simulink model "Arm_core_design_block"  (R2021a)
settings: Solver=VariableStepAuto  StartTime=0.0  StopTime=500  RelTol=1e-3
undefined symbols (not defined in the file or in its folder): AXI4, Lite
libraries: hdlBasic x907, xbsIndex_r4 x1
(part 3 of 7)

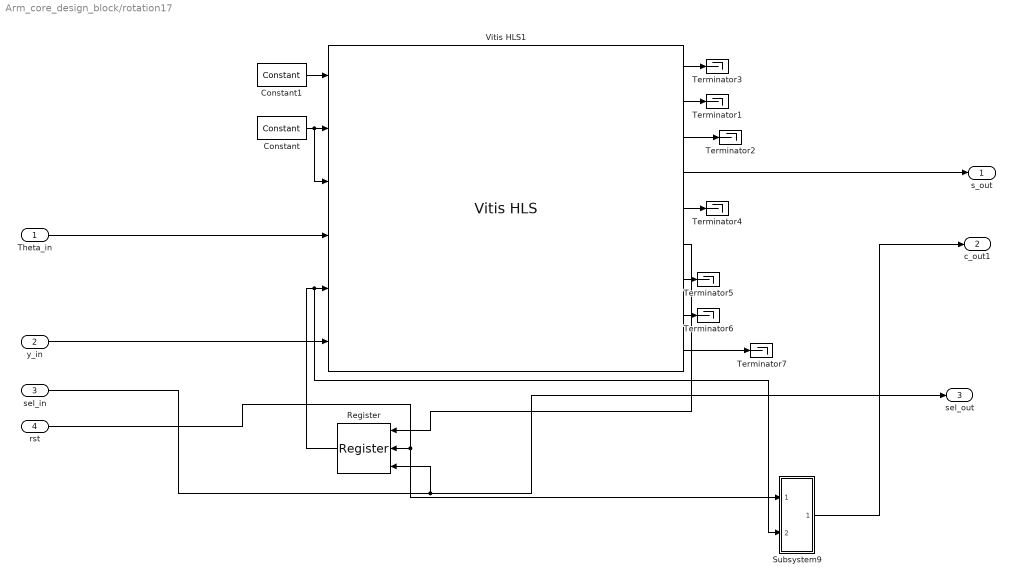
== system Arm_core_design_block/rotation17 ==
  Theta_in : Inport
  y_in : Inport  Port=2
  sel_in : Inport  Port=3
  rst : Inport  Port=4
  Constant : hdlBasic/Constant  const=1.0  gui_display_data_type=Boolean  arith_type=Boolean  n_bits=16  bin_pt=14  preci_type=Single  exp_width=8  frac_width=24  explicit_period=off  period=1  XmcBlockStatus=1  maskContainerNames=tabcontainer1  block_type=constant  block_config=sysgen:Constant_config
  Constant1 : hdlBasic/Constant  const=0  gui_display_data_type=Boolean  arith_type=Boolean  n_bits=16  bin_pt=14  preci_type=Single  exp_width=8  frac_width=24  explicit_period=off  period=1  XmcBlockStatus=1  maskContainerNames=tabcontainer1  block_type=constant  block_config=sysgen:Constant_config
  Register : hdlBasic/Register  init=0  rst=on  en=on  XmcBlockStatus=1  maskContainerNames=tabcontainer1  block_type=register  block_config=sysgen:Register_config
  Subsystem9 : Subsystem
  Terminator{1..7} (7 alike) : Terminator
  Vitis HLS1 : hdlBasic/Vitis HLS  anytable='.\cordic_proj5\solution1'  fast_sim=off  display_datatype=off  rate_propagation_method=Simulink system period  model_file_path=''  latency=1  block_type=vitis_hls
      settings: infoedit=This block allows including C,C++ and SystemC source files in System Generator for DSP designs.
  s_out : Outport
  c_out1 : Outport  Port=2
  sel_out : Outport  Port=3
  wires:
  Constant1/1 -> Vitis HLS1/1
  Vitis HLS1/6 -> Register/1
  y_in/1 -> Vitis HLS1/6
  Constant/1 -> Vitis HLS1/3, Vitis HLS1/2
  Vitis HLS1/4 -> s_out/1
  Theta_in/1 -> Vitis HLS1/4
  sel_in/1 -> sel_out/1, Register/3
  Vitis HLS1/1 -> Terminator3/1
  Vitis HLS1/2 -> Terminator1/1
  Vitis HLS1/3 -> Terminator2/1
  Vitis HLS1/5 -> Terminator4/1
  Vitis HLS1/7 -> Terminator5/1
  Vitis HLS1/8 -> Terminator6/1
  Vitis HLS1/9 -> Terminator7/1
  Register/1 -> Subsystem9/2(reg_i), Vitis HLS1/5
  rst/1 -> Subsystem9/1(rst), Register/2
  Subsystem9/1(reg_o) -> c_out1/1

== system Arm_core_design_block/rotation19 ==
  Theta_in : Inport
  y_in : Inport  Port=2
  rst : Inport  Port=3
  Constant : hdlBasic/Constant  const=1.0  gui_display_data_type=Boolean  arith_type=Boolean  n_bits=16  bin_pt=14  preci_type=Single  exp_width=8  frac_width=24  explicit_period=off  period=1  XmcBlockStatus=1  maskContainerNames=tabcontainer1  block_type=constant  block_config=sysgen:Constant_config
  Constant1 : hdlBasic/Constant  const=0  gui_display_data_type=Boolean  arith_type=Boolean  n_bits=16  bin_pt=14  preci_type=Single  exp_width=8  frac_width=24  explicit_period=off  period=1  XmcBlockStatus=1  maskContainerNames=tabcontainer1  block_type=constant  block_config=sysgen:Constant_config
  Register : hdlBasic/Register  init=0  rst=on  en=on  XmcBlockStatus=1  maskContainerNames=tabcontainer1  block_type=register  block_config=sysgen:Register_config
  Subsystem9 : Subsystem
  Terminator{1..6} (6 alike) : Terminator
  Vitis HLS1 : hdlBasic/Vitis HLS  anytable='.\cordic_proj5\solution1'  fast_sim=off  display_datatype=off  rate_propagation_method=Simulink system period  model_file_path=''  latency=1  block_type=vitis_hls
      settings: infoedit=This block allows including C,C++ and SystemC source files in System Generator for DSP designs.
  s_out : Outport
  c_out1 : Outport  Port=2
  sel_out : Outport  Port=3
  wires:
  Constant1/1 -> Vitis HLS1/1
  Vitis HLS1/6 -> Register/1
  y_in/1 -> Vitis HLS1/6
  Constant/1 -> Vitis HLS1/3, Vitis HLS1/2
  Vitis HLS1/7 -> sel_out/1, Register/3
  Vitis HLS1/4 -> s_out/1
  Theta_in/1 -> Vitis HLS1/4
  Vitis HLS1/1 -> Terminator3/1
  Vitis HLS1/2 -> Terminator1/1
  Vitis HLS1/5 -> Terminator2/1
  Vitis HLS1/8 -> Terminator5/1
  Vitis HLS1/9 -> Terminator4/1
  Vitis HLS1/3 -> Terminator6/1
  rst/1 -> Subsystem9/1(rst), Register/2
  Register/1 -> Subsystem9/2(reg_i), Vitis HLS1/5
  Subsystem9/1(reg_o) -> c_out1/1

== system Arm_core_design_block/rotation2 ==
  Theta_in : Inport
  y_in : Inport  Port=2
  rst : Inport  Port=3
  Constant : hdlBasic/Constant  const=1.0  gui_display_data_type=Boolean  arith_type=Boolean  n_bits=16  bin_pt=14  preci_type=Single  exp_width=8  frac_width=24  explicit_period=off  period=1  XmcBlockStatus=1  maskContainerNames=tabcontainer1  block_type=constant  block_config=sysgen:Constant_config
  Constant1 : hdlBasic/Constant  const=0  gui_display_data_type=Boolean  arith_type=Boolean  n_bits=16  bin_pt=14  preci_type=Single  exp_width=8  frac_width=24  explicit_period=off  period=1  XmcBlockStatus=1  maskContainerNames=tabcontainer1  block_type=constant  block_config=sysgen:Constant_config
  Register : hdlBasic/Register  init=0  rst=on  en=on  XmcBlockStatus=1  maskContainerNames=tabcontainer1  block_type=register  block_config=sysgen:Register_config
  Terminator{1..6} (6 alike) : Terminator
  Vitis HLS1 : hdlBasic/Vitis HLS  anytable='.\cordic_proj5\solution1'  fast_sim=off  display_datatype=off  rate_propagation_method=Simulink system period  model_file_path=''  latency=1  block_type=vitis_hls
      settings: infoedit=This block allows including C,C++ and SystemC source files in System Generator for DSP designs.
  s_out : Outport
  c_out1 : Outport  Port=2
  sel_out : Outport  Port=3
  wires:
  Constant1/1 -> Vitis HLS1/1
  Vitis HLS1/6 -> Register/1
  y_in/1 -> Vitis HLS1/6
  Constant/1 -> Vitis HLS1/3, Vitis HLS1/2
  Vitis HLS1/7 -> sel_out/1, Register/3
  Vitis HLS1/4 -> s_out/1
  Theta_in/1 -> Vitis HLS1/4
  Vitis HLS1/1 -> Terminator3/1
  Vitis HLS1/2 -> Terminator1/1
  Vitis HLS1/5 -> Terminator2/1
  Vitis HLS1/8 -> Terminator5/1
  Vitis HLS1/9 -> Terminator4/1
  Vitis HLS1/3 -> Terminator6/1
  rst/1 -> Register/2
  Register/1 -> c_out1/1, Vitis HLS1/5

== system Arm_core_design_block/rotation3 ==
  Theta_in : Inport
  y_in : Inport  Port=2
  sel_in : Inport  Port=3
  rst : Inport  Port=4
  Constant : hdlBasic/Constant  const=1.0  gui_display_data_type=Boolean  arith_type=Boolean  n_bits=16  bin_pt=14  preci_type=Single  exp_width=8  frac_width=24  explicit_period=off  period=1  XmcBlockStatus=1  maskContainerNames=tabcontainer1  block_type=constant  block_config=sysgen:Constant_config
  Constant1 : hdlBasic/Constant  const=0  gui_display_data_type=Boolean  arith_type=Boolean  n_bits=16  bin_pt=14  preci_type=Single  exp_width=8  frac_width=24  explicit_period=off  period=1  XmcBlockStatus=1  maskContainerNames=tabcontainer1  block_type=constant  block_config=sysgen:Constant_config
  Register : hdlBasic/Register  init=0  rst=on  en=on  XmcBlockStatus=1  maskContainerNames=tabcontainer1  block_type=register  block_config=sysgen:Register_config
  Terminator{1..7} (7 alike) : Terminator
  Vitis HLS1 : hdlBasic/Vitis HLS  anytable='.\cordic_proj5\solution1'  fast_sim=off  display_datatype=off  rate_propagation_method=Simulink system period  model_file_path=''  latency=1  block_type=vitis_hls
      settings: infoedit=This block allows including C,C++ and SystemC source files in System Generator for DSP designs.
  s_out : Outport
  c_out1 : Outport  Port=2
  wires:
  Constant1/1 -> Vitis HLS1/1
  y_in/1 -> Vitis HLS1/6
  Constant/1 -> Vitis HLS1/3, Vitis HLS1/2
  Vitis HLS1/4 -> s_out/1
  Theta_in/1 -> Vitis HLS1/4
  sel_in/1 -> Register/3
  Vitis HLS1/1 -> Terminator3/1
  Vitis HLS1/2 -> Terminator1/1
  Vitis HLS1/3 -> Terminator2/1
  Vitis HLS1/5 -> Terminator4/1
  Vitis HLS1/7 -> Terminator5/1
  Vitis HLS1/8 -> Terminator6/1
  Vitis HLS1/9 -> Terminator7/1
  rst/1 -> Register/2
  Vitis HLS1/6 -> Register/1
  Register/1 -> c_out1/1, Vitis HLS1/5

== system Arm_core_design_block/rotation4 ==
  Theta_in : Inport
  y_in : Inport  Port=2
  rst : Inport  Port=3
  Constant : hdlBasic/Constant  const=1.0  gui_display_data_type=Boolean  arith_type=Boolean  n_bits=16  bin_pt=14  preci_type=Single  exp_width=8  frac_width=24  explicit_period=off  period=1  XmcBlockStatus=1  maskContainerNames=tabcontainer1  block_type=constant  block_config=sysgen:Constant_config
  Constant1 : hdlBasic/Constant  const=0  gui_display_data_type=Boolean  arith_type=Boolean  n_bits=16  bin_pt=14  preci_type=Single  exp_width=8  frac_width=24  explicit_period=off  period=1  XmcBlockStatus=1  maskContainerNames=tabcontainer1  block_type=constant  block_config=sysgen:Constant_config
  Register : hdlBasic/Register  init=0  rst=on  en=on  XmcBlockStatus=1  maskContainerNames=tabcontainer1  block_type=register  block_config=sysgen:Register_config
  Terminator{1..6} (6 alike) : Terminator
  Vitis HLS1 : hdlBasic/Vitis HLS  anytable='.\cordic_proj5\solution1'  fast_sim=off  display_datatype=off  rate_propagation_method=Simulink system period  model_file_path=''  latency=1  block_type=vitis_hls
      settings: infoedit=This block allows including C,C++ and SystemC source files in System Generator for DSP designs.
  s_out : Outport
  c_out1 : Outport  Port=2
  sel_out : Outport  Port=3
  wires:
  Constant1/1 -> Vitis HLS1/1
  Vitis HLS1/6 -> Register/1
  y_in/1 -> Vitis HLS1/6
  Constant/1 -> Vitis HLS1/3, Vitis HLS1/2
  Vitis HLS1/7 -> sel_out/1, Register/3
  Vitis HLS1/4 -> s_out/1
  Theta_in/1 -> Vitis HLS1/4
  Vitis HLS1/1 -> Terminator3/1
  Vitis HLS1/2 -> Terminator1/1
  Vitis HLS1/5 -> Terminator2/1
  Vitis HLS1/8 -> Terminator5/1
  Vitis HLS1/9 -> Terminator4/1
  Vitis HLS1/3 -> Terminator6/1
  rst/1 -> Register/2
  Register/1 -> c_out1/1, Vitis HLS1/5

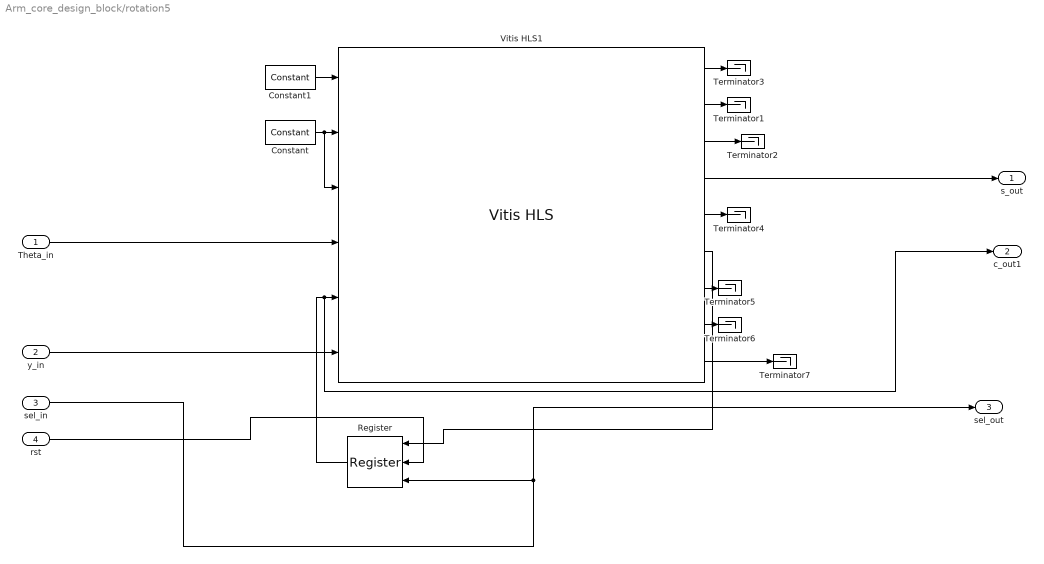
== system Arm_core_design_block/rotation5 ==
  Theta_in : Inport
  y_in : Inport  Port=2
  sel_in : Inport  Port=3
  rst : Inport  Port=4
  Constant : hdlBasic/Constant  const=1.0  gui_display_data_type=Boolean  arith_type=Boolean  n_bits=16  bin_pt=14  preci_type=Single  exp_width=8  frac_width=24  explicit_period=off  period=1  XmcBlockStatus=1  maskContainerNames=tabcontainer1  block_type=constant  block_config=sysgen:Constant_config
  Constant1 : hdlBasic/Constant  const=0  gui_display_data_type=Boolean  arith_type=Boolean  n_bits=16  bin_pt=14  preci_type=Single  exp_width=8  frac_width=24  explicit_period=off  period=1  XmcBlockStatus=1  maskContainerNames=tabcontainer1  block_type=constant  block_config=sysgen:Constant_config
  Register : hdlBasic/Register  init=0  rst=on  en=on  XmcBlockStatus=1  maskContainerNames=tabcontainer1  block_type=register  block_config=sysgen:Register_config
  Terminator{1..7} (7 alike) : Terminator
  Vitis HLS1 : hdlBasic/Vitis HLS  anytable='.\cordic_proj5\solution1'  fast_sim=off  display_datatype=off  rate_propagation_method=Simulink system period  model_file_path=''  latency=1  block_type=vitis_hls
      settings: infoedit=This block allows including C,C++ and SystemC source files in System Generator for DSP designs.
  s_out : Outport
  c_out1 : Outport  Port=2
  sel_out : Outport  Port=3
  wires:
  Constant1/1 -> Vitis HLS1/1
  Vitis HLS1/6 -> Register/1
  y_in/1 -> Vitis HLS1/6
  Constant/1 -> Vitis HLS1/3, Vitis HLS1/2
  Vitis HLS1/4 -> s_out/1
  Theta_in/1 -> Vitis HLS1/4
  sel_in/1 -> sel_out/1, Register/3
  Vitis HLS1/1 -> Terminator3/1
  Vitis HLS1/2 -> Terminator1/1
  Vitis HLS1/3 -> Terminator2/1
  Vitis HLS1/5 -> Terminator4/1
  Vitis HLS1/7 -> Terminator5/1
  Vitis HLS1/8 -> Terminator6/1
  Vitis HLS1/9 -> Terminator7/1
  Register/1 -> c_out1/1, Vitis HLS1/5
  rst/1 -> Register/2

== system Arm_core_design_block/rotation6 ==
  Theta_in : Inport
  y_in : Inport  Port=2
  sel_in : Inport  Port=3
  rst : Inport  Port=4
  Constant : hdlBasic/Constant  const=1.0  gui_display_data_type=Boolean  arith_type=Boolean  n_bits=16  bin_pt=14  preci_type=Single  exp_width=8  frac_width=24  explicit_period=off  period=1  XmcBlockStatus=1  maskContainerNames=tabcontainer1  block_type=constant  block_config=sysgen:Constant_config
  Constant1 : hdlBasic/Constant  const=0  gui_display_data_type=Boolean  arith_type=Boolean  n_bits=16  bin_pt=14  preci_type=Single  exp_width=8  frac_width=24  explicit_period=off  period=1  XmcBlockStatus=1  maskContainerNames=tabcontainer1  block_type=constant  block_config=sysgen:Constant_config
  Register : hdlBasic/Register  init=0  rst=on  en=on  XmcBlockStatus=1  maskContainerNames=tabcontainer1  block_type=register  block_config=sysgen:Register_config
  Register1 : hdlBasic/Register  init=0  rst=on  en=on  XmcBlockStatus=1  maskContainerNames=tabcontainer1  block_type=register  block_config=sysgen:Register_config
  Terminator{1..7} (7 alike) : Terminator
  Vitis HLS1 : hdlBasic/Vitis HLS  anytable='.\cordic_proj5\solution1'  fast_sim=off  display_datatype=off  rate_propagation_method=Simulink system period  model_file_path=''  latency=1  block_type=vitis_hls
      settings: infoedit=This block allows including C,C++ and SystemC source files in System Generator for DSP designs.
  s_out : Outport
  c_out1 : Outport  Port=2
  wires:
  Constant1/1 -> Vitis HLS1/1
  y_in/1 -> Vitis HLS1/6
  Constant/1 -> Vitis HLS1/3, Vitis HLS1/2
  Vitis HLS1/4 -> Register1/1
  Theta_in/1 -> Vitis HLS1/4
  sel_in/1 -> Register1/3, Register/3
  Vitis HLS1/1 -> Terminator3/1
  Vitis HLS1/2 -> Terminator1/1
  Vitis HLS1/3 -> Terminator2/1
  Vitis HLS1/5 -> Terminator4/1
  Vitis HLS1/7 -> Terminator5/1
  Vitis HLS1/8 -> Terminator6/1
  Vitis HLS1/9 -> Terminator7/1
  rst/1 -> Register1/2, Register/2
  Register/1 -> c_out1/1, Vitis HLS1/5
  Vitis HLS1/6 -> Register/1
  Register1/1 -> s_out/1

== system Arm_core_design_block/rotation7 ==
  Theta_in : Inport
  y_in : Inport  Port=2
  rst : Inport  Port=3
  Constant : hdlBasic/Constant  const=1.0  gui_display_data_type=Boolean  arith_type=Boolean  n_bits=16  bin_pt=14  preci_type=Single  exp_width=8  frac_width=24  explicit_period=off  period=1  XmcBlockStatus=1  maskContainerNames=tabcontainer1  block_type=constant  block_config=sysgen:Constant_config
  Constant1 : hdlBasic/Constant  const=0  gui_display_data_type=Boolean  arith_type=Boolean  n_bits=16  bin_pt=14  preci_type=Single  exp_width=8  frac_width=24  explicit_period=off  period=1  XmcBlockStatus=1  maskContainerNames=tabcontainer1  block_type=constant  block_config=sysgen:Constant_config
  Register : hdlBasic/Register  init=0  rst=on  en=on  XmcBlockStatus=1  maskContainerNames=tabcontainer1  block_type=register  block_config=sysgen:Register_config
  Subsystem9 : Subsystem
  Terminator{1..6} (6 alike) : Terminator
  Vitis HLS1 : hdlBasic/Vitis HLS  anytable='.\cordic_proj5\solution1'  fast_sim=off  display_datatype=off  rate_propagation_method=Simulink system period  model_file_path=''  latency=1  block_type=vitis_hls
      settings: infoedit=This block allows including C,C++ and SystemC source files in System Generator for DSP designs.
  s_out : Outport
  c_out1 : Outport  Port=2
  sel_out : Outport  Port=3
  wires:
  Constant1/1 -> Vitis HLS1/1
  Vitis HLS1/6 -> Register/1
  y_in/1 -> Vitis HLS1/6
  Constant/1 -> Vitis HLS1/3, Vitis HLS1/2
  Vitis HLS1/7 -> sel_out/1, Register/3
  Vitis HLS1/4 -> s_out/1
  Theta_in/1 -> Vitis HLS1/4
  Vitis HLS1/1 -> Terminator3/1
  Vitis HLS1/2 -> Terminator1/1
  Vitis HLS1/5 -> Terminator2/1
  Vitis HLS1/8 -> Terminator5/1
  Vitis HLS1/9 -> Terminator4/1
  Vitis HLS1/3 -> Terminator6/1
  rst/1 -> Subsystem9/1(rst), Register/2
  Register/1 -> Subsystem9/2(reg_i), Vitis HLS1/5
  Subsystem9/1(reg_o) -> c_out1/1

== system Arm_core_design_block/rotation8 ==
  Theta_in : Inport
  y_in : Inport  Port=2
  rst : Inport  Port=3
  Constant : hdlBasic/Constant  const=1.0  gui_display_data_type=Boolean  arith_type=Boolean  n_bits=16  bin_pt=14  preci_type=Single  exp_width=8  frac_width=24  explicit_period=off  period=1  XmcBlockStatus=1  maskContainerNames=tabcontainer1  block_type=constant  block_config=sysgen:Constant_config
  Constant1 : hdlBasic/Constant  const=0  gui_display_data_type=Boolean  arith_type=Boolean  n_bits=16  bin_pt=14  preci_type=Single  exp_width=8  frac_width=24  explicit_period=off  period=1  XmcBlockStatus=1  maskContainerNames=tabcontainer1  block_type=constant  block_config=sysgen:Constant_config
  Register : hdlBasic/Register  init=0  rst=on  en=on  XmcBlockStatus=1  maskContainerNames=tabcontainer1  block_type=register  block_config=sysgen:Register_config
  Subsystem9 : Subsystem
  Terminator{1..6} (6 alike) : Terminator
  Vitis HLS1 : hdlBasic/Vitis HLS  anytable='.\cordic_proj5\solution1'  fast_sim=off  display_datatype=off  rate_propagation_method=Simulink system period  model_file_path=''  latency=1  block_type=vitis_hls
      settings: infoedit=This block allows including C,C++ and SystemC source files in System Generator for DSP designs.
  s_out : Outport
  c_out1 : Outport  Port=2
  sel_out : Outport  Port=3
  wires:
  Constant1/1 -> Vitis HLS1/1
  Vitis HLS1/6 -> Register/1
  y_in/1 -> Vitis HLS1/6
  Constant/1 -> Vitis HLS1/3, Vitis HLS1/2
  Vitis HLS1/7 -> sel_out/1, Register/3
  Vitis HLS1/4 -> s_out/1
  Theta_in/1 -> Vitis HLS1/4
  Vitis HLS1/1 -> Terminator3/1
  Vitis HLS1/2 -> Terminator1/1
  Vitis HLS1/5 -> Terminator2/1
  Vitis HLS1/8 -> Terminator5/1
  Vitis HLS1/9 -> Terminator4/1
  Vitis HLS1/3 -> Terminator6/1
  rst/1 -> Subsystem9/1(rst), Register/2
  Register/1 -> Subsystem9/2(reg_i), Vitis HLS1/5
  Subsystem9/1(reg_o) -> c_out1/1

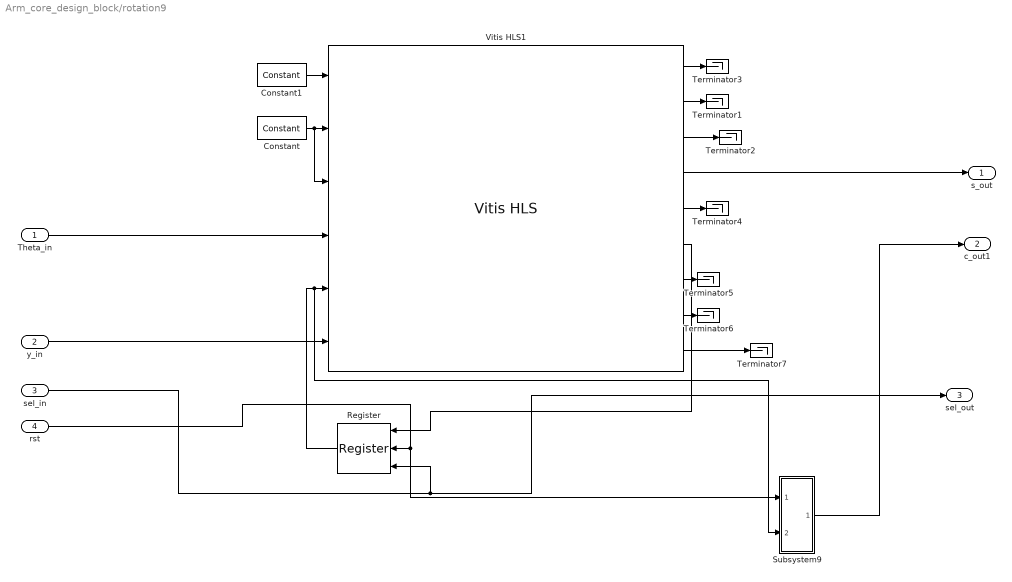
== system Arm_core_design_block/rotation9 ==
  Theta_in : Inport
  y_in : Inport  Port=2
  sel_in : Inport  Port=3
  rst : Inport  Port=4
  Constant : hdlBasic/Constant  const=1.0  gui_display_data_type=Boolean  arith_type=Boolean  n_bits=16  bin_pt=14  preci_type=Single  exp_width=8  frac_width=24  explicit_period=off  period=1  XmcBlockStatus=1  maskContainerNames=tabcontainer1  block_type=constant  block_config=sysgen:Constant_config
  Constant1 : hdlBasic/Constant  const=0  gui_display_data_type=Boolean  arith_type=Boolean  n_bits=16  bin_pt=14  preci_type=Single  exp_width=8  frac_width=24  explicit_period=off  period=1  XmcBlockStatus=1  maskContainerNames=tabcontainer1  block_type=constant  block_config=sysgen:Constant_config
  Register : hdlBasic/Register  init=0  rst=on  en=on  XmcBlockStatus=1  maskContainerNames=tabcontainer1  block_type=register  block_config=sysgen:Register_config
  Subsystem9 : Subsystem
  Terminator{1..7} (7 alike) : Terminator
  Vitis HLS1 : hdlBasic/Vitis HLS  anytable='.\cordic_proj5\solution1'  fast_sim=off  display_datatype=off  rate_propagation_method=Simulink system period  model_file_path=''  latency=1  block_type=vitis_hls
      settings: infoedit=This block allows including C,C++ and SystemC source files in System Generator for DSP designs.
  s_out : Outport
  c_out1 : Outport  Port=2
  sel_out : Outport  Port=3
  wires:
  Constant1/1 -> Vitis HLS1/1
  Vitis HLS1/6 -> Register/1
  y_in/1 -> Vitis HLS1/6
  Constant/1 -> Vitis HLS1/3, Vitis HLS1/2
  Vitis HLS1/4 -> s_out/1
  Theta_in/1 -> Vitis HLS1/4
  sel_in/1 -> sel_out/1, Register/3
  Vitis HLS1/1 -> Terminator3/1
  Vitis HLS1/2 -> Terminator1/1
  Vitis HLS1/3 -> Terminator2/1
  Vitis HLS1/5 -> Terminator4/1
  Vitis HLS1/7 -> Terminator5/1
  Vitis HLS1/8 -> Terminator6/1
  Vitis HLS1/9 -> Terminator7/1
  Register/1 -> Subsystem9/2(reg_i), Vitis HLS1/5
  rst/1 -> Subsystem9/1(rst), Register/2
  Subsystem9/1(reg_o) -> c_out1/1

== system Arm_core_design_block/Subsystem10/Subsystem10 ==
  reg_i : Inport
  Constant1 : hdlBasic/Constant  const=0  gui_display_data_type=Boolean  arith_type=Boolean  n_bits=16  bin_pt=1  preci_type=Single  exp_width=8  frac_width=24  explicit_period=off  period=1  XmcBlockStatus=1  maskContainerNames=tabcontainer1  block_type=constant  block_config=sysgen:Constant_config
  Mux1 : hdlBasic/Mux  inputs=2  en=off  latency=1  precision=Full  arith_type=Unsigned  n_bits=16  bin_pt=14  quantization=Truncate  overflow=Wrap  XmcBlockStatus=1  maskContainerNames=tabcontainer1  block_type=mux  block_config=sysgen:Mux_config
  Register2 : hdlBasic/Register  init=0  rst=off  en=off  XmcBlockStatus=1  maskContainerNames=tabcontainer1  block_type=register  block_config=sysgen:Register_config
  reg_o : Outport
  wires:
  reg_i/1 -> Register2/1, Mux1/2
  Mux1/1 -> reg_o/1
  Constant1/1 -> Mux1/3
  Register2/1 -> Mux1/1

== system Arm_core_design_block/Subsystem10/Subsystem11 ==
  rst : Inport
  reg_i : Inport  Port=2
  Absolute1 : hdlBasic/Absolute  precision=User Defined  arith_type="Signed  (2's comp)"  n_bits=16  bin_pt=13  quantization=Truncate  overflow=Saturate  en=off  latency=0  XmcBlockStatus=1  maskContainerNames=tabcontainer1  block_type=abs  block_config=sysgen:Abs_config
  Accumulator1 : hdlBasic/Accumulator  operation=Add  n_bits=16  overflow=Wrap  scale=1  rst=on  hasbypass=off  en=on  latency=1  msb_inp=100  msb=100  lsb=-100  use_behavioral_HDL=on  implementation=Fabric  XmcBlockStatus=1  maskContainerNames=group3  block_type=accum  block_config=sysgen:Accum_config
  Constant4 : hdlBasic/Constant  const=0.05  gui_display_data_type=Fixed-point  arith_type=Signed (2's comp)  n_bits=16  bin_pt=14  preci_type=Single  exp_width=8  frac_width=24  explicit_period=off  period=1  XmcBlockStatus=1  maskContainerNames=tabcontainer1  block_type=constant  block_config=sysgen:Constant_config
  Constant5 : hdlBasic/Constant  const=1  gui_display_data_type=Fixed-point  arith_type=Unsigned  n_bits=16  bin_pt=1  preci_type=Single  exp_width=8  frac_width=24  explicit_period=off  period=1  XmcBlockStatus=1  maskContainerNames=tabcontainer1  block_type=constant  block_config=sysgen:Constant_config
  Constant6 : hdlBasic/Constant  const=0  gui_display_data_type=Fixed-point  arith_type=Unsigned  n_bits=16  bin_pt=1  preci_type=Single  exp_width=8  frac_width=24  explicit_period=off  period=1  XmcBlockStatus=1  maskContainerNames=tabcontainer1  block_type=constant  block_config=sysgen:Constant_config
  Constant7 : hdlBasic/Constant  const=0  gui_display_data_type=Boolean  arith_type=Boolean  n_bits=16  bin_pt=1  preci_type=Single  exp_width=8  frac_width=24  explicit_period=off  period=1  XmcBlockStatus=1  maskContainerNames=tabcontainer1  block_type=constant  block_config=sysgen:Constant_config
  Mux1 : hdlBasic/Mux  inputs=2  en=off  latency=0  precision=Full  arith_type=Unsigned  n_bits=16  bin_pt=14  quantization=Truncate  overflow=Wrap  XmcBlockStatus=1  maskContainerNames=tabcontainer1  block_type=mux  block_config=sysgen:Mux_config
  Register1 : hdlBasic/Register  init=0  rst=on  en=on  XmcBlockStatus=1  maskContainerNames=tabcontainer1  block_type=register  block_config=sysgen:Register_config
  Relational2 : hdlBasic/Relational  mode=a>b  op_type=Bool  en=off  latency=0  XmcBlockStatus=1  maskContainerNames=tabcontainer1  block_type=relational  block_config=sysgen:Relational_config
  Relational3 : hdlBasic/Relational  mode=a>b  op_type=Bool  en=off  latency=0  XmcBlockStatus=1  maskContainerNames=tabcontainer1  block_type=relational  block_config=sysgen:Relational_config
  reg_o : Outport
  wires:
  Constant5/1 -> Accumulator1/1
  Relational2/1 -> Mux1/2
  Constant7/1 -> Mux1/3
  reg_i/1 -> Absolute1/1, Register1/1
  rst/1 -> Register1/2, Accumulator1/2
  Constant6/1 -> Relational3/2
  Accumulator1/1 -> Relational3/1
  Relational3/1 -> Mux1/1
  Mux1/1 -> Register1/3, Accumulator1/3
  Absolute1/1 -> Relational2/1
  Constant4/1 -> Relational2/2
  Register1/1 -> reg_o/1

== system Arm_core_design_block/Subsystem10/Subsystem12 ==
  rst : Inport
  reg_i : Inport  Port=2
  Absolute1 : hdlBasic/Absolute  precision=User Defined  arith_type="Signed  (2's comp)"  n_bits=16  bin_pt=13  quantization=Truncate  overflow=Saturate  en=off  latency=0  XmcBlockStatus=1  maskContainerNames=tabcontainer1  block_type=abs  block_config=sysgen:Abs_config
  Accumulator1 : hdlBasic/Accumulator  operation=Add  n_bits=16  overflow=Wrap  scale=1  rst=on  hasbypass=off  en=on  latency=1  msb_inp=100  msb=100  lsb=-100  use_behavioral_HDL=on  implementation=Fabric  XmcBlockStatus=1  maskContainerNames=group3  block_type=accum  block_config=sysgen:Accum_config
  Constant4 : hdlBasic/Constant  const=0.05  gui_display_data_type=Fixed-point  arith_type=Signed (2's comp)  n_bits=16  bin_pt=14  preci_type=Single  exp_width=8  frac_width=24  explicit_period=off  period=1  XmcBlockStatus=1  maskContainerNames=tabcontainer1  block_type=constant  block_config=sysgen:Constant_config
  Constant5 : hdlBasic/Constant  const=1  gui_display_data_type=Fixed-point  arith_type=Unsigned  n_bits=16  bin_pt=1  preci_type=Single  exp_width=8  frac_width=24  explicit_period=off  period=1  XmcBlockStatus=1  maskContainerNames=tabcontainer1  block_type=constant  block_config=sysgen:Constant_config
  Constant6 : hdlBasic/Constant  const=0  gui_display_data_type=Fixed-point  arith_type=Unsigned  n_bits=16  bin_pt=1  preci_type=Single  exp_width=8  frac_width=24  explicit_period=off  period=1  XmcBlockStatus=1  maskContainerNames=tabcontainer1  block_type=constant  block_config=sysgen:Constant_config
  Constant7 : hdlBasic/Constant  const=0  gui_display_data_type=Boolean  arith_type=Boolean  n_bits=16  bin_pt=1  preci_type=Single  exp_width=8  frac_width=24  explicit_period=off  period=1  XmcBlockStatus=1  maskContainerNames=tabcontainer1  block_type=constant  block_config=sysgen:Constant_config
  Mux1 : hdlBasic/Mux  inputs=2  en=off  latency=0  precision=Full  arith_type=Unsigned  n_bits=16  bin_pt=14  quantization=Truncate  overflow=Wrap  XmcBlockStatus=1  maskContainerNames=tabcontainer1  block_type=mux  block_config=sysgen:Mux_config
  Register1 : hdlBasic/Register  init=0  rst=on  en=on  XmcBlockStatus=1  maskContainerNames=tabcontainer1  block_type=register  block_config=sysgen:Register_config
  Relational2 : hdlBasic/Relational  mode=a>b  op_type=Bool  en=off  latency=0  XmcBlockStatus=1  maskContainerNames=tabcontainer1  block_type=relational  block_config=sysgen:Relational_config
  Relational3 : hdlBasic/Relational  mode=a>b  op_type=Bool  en=off  latency=0  XmcBlockStatus=1  maskContainerNames=tabcontainer1  block_type=relational  block_config=sysgen:Relational_config
  reg_o : Outport
  wires:
  Constant5/1 -> Accumulator1/1
  Relational2/1 -> Mux1/2
  Constant7/1 -> Mux1/3
  reg_i/1 -> Absolute1/1, Register1/1
  rst/1 -> Register1/2, Accumulator1/2
  Constant6/1 -> Relational3/2
  Accumulator1/1 -> Relational3/1
  Relational3/1 -> Mux1/1
  Mux1/1 -> Register1/3, Accumulator1/3
  Absolute1/1 -> Relational2/1
  Constant4/1 -> Relational2/2
  Register1/1 -> reg_o/1

== system Arm_core_design_block/Subsystem10/Subsystem13 ==
  rst : Inport
  reg_i : Inport  Port=2
  Absolute1 : hdlBasic/Absolute  precision=User Defined  arith_type="Signed  (2's comp)"  n_bits=16  bin_pt=13  quantization=Truncate  overflow=Saturate  en=off  latency=0  XmcBlockStatus=1  maskContainerNames=tabcontainer1  block_type=abs  block_config=sysgen:Abs_config
  Accumulator1 : hdlBasic/Accumulator  operation=Add  n_bits=16  overflow=Wrap  scale=1  rst=on  hasbypass=off  en=on  latency=1  msb_inp=100  msb=100  lsb=-100  use_behavioral_HDL=on  implementation=Fabric  XmcBlockStatus=1  maskContainerNames=group3  block_type=accum  block_config=sysgen:Accum_config
  Constant4 : hdlBasic/Constant  const=0  gui_display_data_type=Fixed-point  arith_type=Signed (2's comp)  n_bits=16  bin_pt=14  preci_type=Single  exp_width=8  frac_width=24  explicit_period=off  period=1  XmcBlockStatus=1  maskContainerNames=tabcontainer1  block_type=constant  block_config=sysgen:Constant_config
  Constant5 : hdlBasic/Constant  const=1  gui_display_data_type=Fixed-point  arith_type=Unsigned  n_bits=16  bin_pt=1  preci_type=Single  exp_width=8  frac_width=24  explicit_period=off  period=1  XmcBlockStatus=1  maskContainerNames=tabcontainer1  block_type=constant  block_config=sysgen:Constant_config
  Constant6 : hdlBasic/Constant  const=0  gui_display_data_type=Fixed-point  arith_type=Unsigned  n_bits=16  bin_pt=1  preci_type=Single  exp_width=8  frac_width=24  explicit_period=off  period=1  XmcBlockStatus=1  maskContainerNames=tabcontainer1  block_type=constant  block_config=sysgen:Constant_config
  Constant7 : hdlBasic/Constant  const=0  gui_display_data_type=Boolean  arith_type=Boolean  n_bits=16  bin_pt=1  preci_type=Single  exp_width=8  frac_width=24  explicit_period=off  period=1  XmcBlockStatus=1  maskContainerNames=tabcontainer1  block_type=constant  block_config=sysgen:Constant_config
  Mux1 : hdlBasic/Mux  inputs=2  en=off  latency=0  precision=Full  arith_type=Unsigned  n_bits=16  bin_pt=14  quantization=Truncate  overflow=Wrap  XmcBlockStatus=1  maskContainerNames=tabcontainer1  block_type=mux  block_config=sysgen:Mux_config
  Register1 : hdlBasic/Register  init=0  rst=on  en=on  XmcBlockStatus=1  maskContainerNames=tabcontainer1  block_type=register  block_config=sysgen:Register_config
  Relational2 : hdlBasic/Relational  mode=a>b  op_type=Bool  en=off  latency=0  XmcBlockStatus=1  maskContainerNames=tabcontainer1  block_type=relational  block_config=sysgen:Relational_config
  Relational3 : hdlBasic/Relational  mode=a>b  op_type=Bool  en=off  latency=0  XmcBlockStatus=1  maskContainerNames=tabcontainer1  block_type=relational  block_config=sysgen:Relational_config
  reg_o : Outport
  wires:
  Constant5/1 -> Accumulator1/1
  Relational2/1 -> Mux1/2
  Constant7/1 -> Mux1/3
  reg_i/1 -> Absolute1/1, Register1/1
  rst/1 -> Register1/2, Accumulator1/2
  Constant6/1 -> Relational3/2
  Accumulator1/1 -> Relational3/1
  Relational3/1 -> Mux1/1
  Mux1/1 -> Register1/3, Accumulator1/3
  Absolute1/1 -> Relational2/1
  Constant4/1 -> Relational2/2
  Register1/1 -> reg_o/1

== system Arm_core_design_block/Subsystem10/Subsystem14 ==
  rst : Inport
  reg_i : Inport  Port=2
  Absolute1 : hdlBasic/Absolute  precision=User Defined  arith_type="Signed  (2's comp)"  n_bits=16  bin_pt=13  quantization=Truncate  overflow=Saturate  en=off  latency=0  XmcBlockStatus=1  maskContainerNames=tabcontainer1  block_type=abs  block_config=sysgen:Abs_config
  Accumulator1 : hdlBasic/Accumulator  operation=Add  n_bits=16  overflow=Wrap  scale=1  rst=on  hasbypass=off  en=on  latency=1  msb_inp=100  msb=100  lsb=-100  use_behavioral_HDL=on  implementation=Fabric  XmcBlockStatus=1  maskContainerNames=group3  block_type=accum  block_config=sysgen:Accum_config
  Constant4 : hdlBasic/Constant  const=0.05  gui_display_data_type=Fixed-point  arith_type=Signed (2's comp)  n_bits=16  bin_pt=14  preci_type=Single  exp_width=8  frac_width=24  explicit_period=off  period=1  XmcBlockStatus=1  maskContainerNames=tabcontainer1  block_type=constant  block_config=sysgen:Constant_config
  Constant5 : hdlBasic/Constant  const=1  gui_display_data_type=Fixed-point  arith_type=Unsigned  n_bits=16  bin_pt=1  preci_type=Single  exp_width=8  frac_width=24  explicit_period=off  period=1  XmcBlockStatus=1  maskContainerNames=tabcontainer1  block_type=constant  block_config=sysgen:Constant_config
  Constant6 : hdlBasic/Constant  const=0  gui_display_data_type=Fixed-point  arith_type=Unsigned  n_bits=16  bin_pt=1  preci_type=Single  exp_width=8  frac_width=24  explicit_period=off  period=1  XmcBlockStatus=1  maskContainerNames=tabcontainer1  block_type=constant  block_config=sysgen:Constant_config
  Constant7 : hdlBasic/Constant  const=0  gui_display_data_type=Boolean  arith_type=Boolean  n_bits=16  bin_pt=1  preci_type=Single  exp_width=8  frac_width=24  explicit_period=off  period=1  XmcBlockStatus=1  maskContainerNames=tabcontainer1  block_type=constant  block_config=sysgen:Constant_config
  Mux1 : hdlBasic/Mux  inputs=2  en=off  latency=0  precision=Full  arith_type=Unsigned  n_bits=16  bin_pt=14  quantization=Truncate  overflow=Wrap  XmcBlockStatus=1  maskContainerNames=tabcontainer1  block_type=mux  block_config=sysgen:Mux_config
  Register1 : hdlBasic/Register  init=0  rst=on  en=on  XmcBlockStatus=1  maskContainerNames=tabcontainer1  block_type=register  block_config=sysgen:Register_config
  Relational2 : hdlBasic/Relational  mode=a>b  op_type=Bool  en=off  latency=0  XmcBlockStatus=1  maskContainerNames=tabcontainer1  block_type=relational  block_config=sysgen:Relational_config
  Relational3 : hdlBasic/Relational  mode=a>b  op_type=Bool  en=off  latency=0  XmcBlockStatus=1  maskContainerNames=tabcontainer1  block_type=relational  block_config=sysgen:Relational_config
  reg_o : Outport
  wires:
  Constant5/1 -> Accumulator1/1
  Relational2/1 -> Mux1/2
  Constant7/1 -> Mux1/3
  reg_i/1 -> Absolute1/1, Register1/1
  rst/1 -> Register1/2, Accumulator1/2
  Constant6/1 -> Relational3/2
  Accumulator1/1 -> Relational3/1
  Relational3/1 -> Mux1/1
  Mux1/1 -> Register1/3, Accumulator1/3
  Absolute1/1 -> Relational2/1
  Constant4/1 -> Relational2/2
  Register1/1 -> reg_o/1

== system Arm_core_design_block/Subsystem10/Subsystem3 ==
  rst : Inport
  in_pulse : Inport  Port=2
  Accumulator2 : hdlBasic/Accumulator  operation=Add  n_bits=3  overflow=Wrap  scale=1  rst=on  hasbypass=off  en=on  latency=1  msb_inp=100  msb=100  lsb=-100  use_behavioral_HDL=on  implementation=Fabric  XmcBlockStatus=1  maskContainerNames=group3  block_type=accum  block_config=sysgen:Accum_config
  Constant1 : hdlBasic/Constant  const=1  gui_display_data_type=Fixed-point  arith_type=Unsigned  n_bits=3  bin_pt=0  preci_type=Single  exp_width=8  frac_width=24  explicit_period=off  period=1  XmcBlockStatus=1  maskContainerNames=tabcontainer1  block_type=constant  block_config=sysgen:Constant_config
  Constant2 : hdlBasic/Constant  const=0  gui_display_data_type=Fixed-point  arith_type=Unsigned  n_bits=3  bin_pt=0  preci_type=Single  exp_width=8  frac_width=24  explicit_period=off  period=1  XmcBlockStatus=1  maskContainerNames=tabcontainer1  block_type=constant  block_config=sysgen:Constant_config
  Delay : hdlBasic/Delay  rst=off  en=off  latency=25  reg_retiming=off  XmcBlockStatus=1  maskContainerNames=group1  block_type=delay  block_config=sysgen:Delay_config
  Delay1 : hdlBasic/Delay  rst=off  en=off  latency=25  reg_retiming=off  XmcBlockStatus=1  maskContainerNames=group1  block_type=delay  block_config=sysgen:Delay_config
  Delay2 : hdlBasic/Delay  rst=off  en=off  latency=25  reg_retiming=off  XmcBlockStatus=1  maskContainerNames=group1  block_type=delay  block_config=sysgen:Delay_config
  Delay3 : hdlBasic/Delay  rst=off  en=off  latency=1  reg_retiming=off  XmcBlockStatus=1  maskContainerNames=group1  block_type=delay  block_config=sysgen:Delay_config
  Logical : hdlBasic/Logical  logical_function=OR  inputs=4  en=off  latency=0  precision=Full  arith_type=Unsigned  n_bits=16  bin_pt=0  align_bp=on  overflow=[]  quantization=[]  XmcBlockStatus=1  maskContainerNames=tabcontainer1  block_type=logical  block_config=sysgen:Logical_config
  Mux : hdlBasic/Mux  inputs=2  en=off  latency=0  precision=Full  arith_type=Unsigned  n_bits=16  bin_pt=14  quantization=Truncate  overflow=Wrap  XmcBlockStatus=1  maskContainerNames=tabcontainer1  block_type=mux  block_config=sysgen:Mux_config
  reg_o : Outport
  wires:
  in_pulse/1 -> Delay/1, Logical/1
  rst/1 -> Accumulator2/2
  Constant1/1 -> Accumulator2/1
  Delay/1 -> Delay1/1, Logical/2
  Logical/1 -> Accumulator2/3, Delay3/1
  Accumulator2/1 -> Mux/3
  Delay2/1 -> Logical/4
  Delay1/1 -> Delay2/1, Logical/3
  Constant2/1 -> Mux/2
  Mux/1 -> reg_o/1
  Delay3/1 -> Mux/1

== system Arm_core_design_block/Subsystem11/Subsystem10 ==
  reg_i : Inport
  Constant1 : hdlBasic/Constant  const=0  gui_display_data_type=Boolean  arith_type=Boolean  n_bits=16  bin_pt=1  preci_type=Single  exp_width=8  frac_width=24  explicit_period=off  period=1  XmcBlockStatus=1  maskContainerNames=tabcontainer1  block_type=constant  block_config=sysgen:Constant_config
  Mux1 : hdlBasic/Mux  inputs=2  en=off  latency=1  precision=Full  arith_type=Unsigned  n_bits=16  bin_pt=14  quantization=Truncate  overflow=Wrap  XmcBlockStatus=1  maskContainerNames=tabcontainer1  block_type=mux  block_config=sysgen:Mux_config
  Register2 : hdlBasic/Register  init=0  rst=off  en=off  XmcBlockStatus=1  maskContainerNames=tabcontainer1  block_type=register  block_config=sysgen:Register_config
  reg_o : Outport
  wires:
  reg_i/1 -> Register2/1, Mux1/2
  Mux1/1 -> reg_o/1
  Constant1/1 -> Mux1/3
  Register2/1 -> Mux1/1

== system Arm_core_design_block/Subsystem11/Subsystem11 ==
  rst : Inport
  reg_i : Inport  Port=2
  Absolute1 : hdlBasic/Absolute  precision=User Defined  arith_type="Signed  (2's comp)"  n_bits=16  bin_pt=13  quantization=Truncate  overflow=Saturate  en=off  latency=0  XmcBlockStatus=1  maskContainerNames=tabcontainer1  block_type=abs  block_config=sysgen:Abs_config
  Accumulator1 : hdlBasic/Accumulator  operation=Add  n_bits=16  overflow=Wrap  scale=1  rst=on  hasbypass=off  en=on  latency=1  msb_inp=100  msb=100  lsb=-100  use_behavioral_HDL=on  implementation=Fabric  XmcBlockStatus=1  maskContainerNames=group3  block_type=accum  block_config=sysgen:Accum_config
  Constant4 : hdlBasic/Constant  const=0.05  gui_display_data_type=Fixed-point  arith_type=Signed (2's comp)  n_bits=16  bin_pt=14  preci_type=Single  exp_width=8  frac_width=24  explicit_period=off  period=1  XmcBlockStatus=1  maskContainerNames=tabcontainer1  block_type=constant  block_config=sysgen:Constant_config
  Constant5 : hdlBasic/Constant  const=1  gui_display_data_type=Fixed-point  arith_type=Unsigned  n_bits=16  bin_pt=1  preci_type=Single  exp_width=8  frac_width=24  explicit_period=off  period=1  XmcBlockStatus=1  maskContainerNames=tabcontainer1  block_type=constant  block_config=sysgen:Constant_config
  Constant6 : hdlBasic/Constant  const=0  gui_display_data_type=Fixed-point  arith_type=Unsigned  n_bits=16  bin_pt=1  preci_type=Single  exp_width=8  frac_width=24  explicit_period=off  period=1  XmcBlockStatus=1  maskContainerNames=tabcontainer1  block_type=constant  block_config=sysgen:Constant_config
  Constant7 : hdlBasic/Constant  const=0  gui_display_data_type=Boolean  arith_type=Boolean  n_bits=16  bin_pt=1  preci_type=Single  exp_width=8  frac_width=24  explicit_period=off  period=1  XmcBlockStatus=1  maskContainerNames=tabcontainer1  block_type=constant  block_config=sysgen:Constant_config
  Mux1 : hdlBasic/Mux  inputs=2  en=off  latency=0  precision=Full  arith_type=Unsigned  n_bits=16  bin_pt=14  quantization=Truncate  overflow=Wrap  XmcBlockStatus=1  maskContainerNames=tabcontainer1  block_type=mux  block_config=sysgen:Mux_config
  Register1 : hdlBasic/Register  init=0  rst=on  en=on  XmcBlockStatus=1  maskContainerNames=tabcontainer1  block_type=register  block_config=sysgen:Register_config
  Relational2 : hdlBasic/Relational  mode=a>b  op_type=Bool  en=off  latency=0  XmcBlockStatus=1  maskContainerNames=tabcontainer1  block_type=relational  block_config=sysgen:Relational_config
  Relational3 : hdlBasic/Relational  mode=a>b  op_type=Bool  en=off  latency=0  XmcBlockStatus=1  maskContainerNames=tabcontainer1  block_type=relational  block_config=sysgen:Relational_config
  reg_o : Outport
  wires:
  Constant5/1 -> Accumulator1/1
  Relational2/1 -> Mux1/2
  Constant7/1 -> Mux1/3
  reg_i/1 -> Absolute1/1, Register1/1
  rst/1 -> Register1/2, Accumulator1/2
  Constant6/1 -> Relational3/2
  Accumulator1/1 -> Relational3/1
  Relational3/1 -> Mux1/1
  Mux1/1 -> Register1/3, Accumulator1/3
  Absolute1/1 -> Relational2/1
  Constant4/1 -> Relational2/2
  Register1/1 -> reg_o/1

== system Arm_core_design_block/Subsystem11/Subsystem12 ==
  rst : Inport
  reg_i : Inport  Port=2
  Absolute1 : hdlBasic/Absolute  precision=User Defined  arith_type="Signed  (2's comp)"  n_bits=16  bin_pt=13  quantization=Truncate  overflow=Saturate  en=off  latency=0  XmcBlockStatus=1  maskContainerNames=tabcontainer1  block_type=abs  block_config=sysgen:Abs_config
  Accumulator1 : hdlBasic/Accumulator  operation=Add  n_bits=16  overflow=Wrap  scale=1  rst=on  hasbypass=off  en=on  latency=1  msb_inp=100  msb=100  lsb=-100  use_behavioral_HDL=on  implementation=Fabric  XmcBlockStatus=1  maskContainerNames=group3  block_type=accum  block_config=sysgen:Accum_config
  Constant4 : hdlBasic/Constant  const=0.05  gui_display_data_type=Fixed-point  arith_type=Signed (2's comp)  n_bits=16  bin_pt=14  preci_type=Single  exp_width=8  frac_width=24  explicit_period=off  period=1  XmcBlockStatus=1  maskContainerNames=tabcontainer1  block_type=constant  block_config=sysgen:Constant_config
  Constant5 : hdlBasic/Constant  const=1  gui_display_data_type=Fixed-point  arith_type=Unsigned  n_bits=16  bin_pt=1  preci_type=Single  exp_width=8  frac_width=24  explicit_period=off  period=1  XmcBlockStatus=1  maskContainerNames=tabcontainer1  block_type=constant  block_config=sysgen:Constant_config
  Constant6 : hdlBasic/Constant  const=0  gui_display_data_type=Fixed-point  arith_type=Unsigned  n_bits=16  bin_pt=1  preci_type=Single  exp_width=8  frac_width=24  explicit_period=off  period=1  XmcBlockStatus=1  maskContainerNames=tabcontainer1  block_type=constant  block_config=sysgen:Constant_config
  Constant7 : hdlBasic/Constant  const=0  gui_display_data_type=Boolean  arith_type=Boolean  n_bits=16  bin_pt=1  preci_type=Single  exp_width=8  frac_width=24  explicit_period=off  period=1  XmcBlockStatus=1  maskContainerNames=tabcontainer1  block_type=constant  block_config=sysgen:Constant_config
  Mux1 : hdlBasic/Mux  inputs=2  en=off  latency=0  precision=Full  arith_type=Unsigned  n_bits=16  bin_pt=14  quantization=Truncate  overflow=Wrap  XmcBlockStatus=1  maskContainerNames=tabcontainer1  block_type=mux  block_config=sysgen:Mux_config
  Register1 : hdlBasic/Register  init=0  rst=on  en=on  XmcBlockStatus=1  maskContainerNames=tabcontainer1  block_type=register  block_config=sysgen:Register_config
  Relational2 : hdlBasic/Relational  mode=a>b  op_type=Bool  en=off  latency=0  XmcBlockStatus=1  maskContainerNames=tabcontainer1  block_type=relational  block_config=sysgen:Relational_config
  Relational3 : hdlBasic/Relational  mode=a>b  op_type=Bool  en=off  latency=0  XmcBlockStatus=1  maskContainerNames=tabcontainer1  block_type=relational  block_config=sysgen:Relational_config
  reg_o : Outport
  wires:
  Constant5/1 -> Accumulator1/1
  Relational2/1 -> Mux1/2
  Constant7/1 -> Mux1/3
  reg_i/1 -> Absolute1/1, Register1/1
  rst/1 -> Register1/2, Accumulator1/2
  Constant6/1 -> Relational3/2
  Accumulator1/1 -> Relational3/1
  Relational3/1 -> Mux1/1
  Mux1/1 -> Register1/3, Accumulator1/3
  Absolute1/1 -> Relational2/1
  Constant4/1 -> Relational2/2
  Register1/1 -> reg_o/1

== system Arm_core_design_block/Subsystem11/Subsystem13 ==
  rst : Inport
  reg_i : Inport  Port=2
  Absolute1 : hdlBasic/Absolute  precision=User Defined  arith_type="Signed  (2's comp)"  n_bits=16  bin_pt=13  quantization=Truncate  overflow=Saturate  en=off  latency=0  XmcBlockStatus=1  maskContainerNames=tabcontainer1  block_type=abs  block_config=sysgen:Abs_config
  Accumulator1 : hdlBasic/Accumulator  operation=Add  n_bits=16  overflow=Wrap  scale=1  rst=on  hasbypass=off  en=on  latency=1  msb_inp=100  msb=100  lsb=-100  use_behavioral_HDL=on  implementation=Fabric  XmcBlockStatus=1  maskContainerNames=group3  block_type=accum  block_config=sysgen:Accum_config
  Constant4 : hdlBasic/Constant  const=0  gui_display_data_type=Fixed-point  arith_type=Signed (2's comp)  n_bits=16  bin_pt=14  preci_type=Single  exp_width=8  frac_width=24  explicit_period=off  period=1  XmcBlockStatus=1  maskContainerNames=tabcontainer1  block_type=constant  block_config=sysgen:Constant_config
  Constant5 : hdlBasic/Constant  const=1  gui_display_data_type=Fixed-point  arith_type=Unsigned  n_bits=16  bin_pt=1  preci_type=Single  exp_width=8  frac_width=24  explicit_period=off  period=1  XmcBlockStatus=1  maskContainerNames=tabcontainer1  block_type=constant  block_config=sysgen:Constant_config
  Constant6 : hdlBasic/Constant  const=0  gui_display_data_type=Fixed-point  arith_type=Unsigned  n_bits=16  bin_pt=1  preci_type=Single  exp_width=8  frac_width=24  explicit_period=off  period=1  XmcBlockStatus=1  maskContainerNames=tabcontainer1  block_type=constant  block_config=sysgen:Constant_config
  Constant7 : hdlBasic/Constant  const=0  gui_display_data_type=Boolean  arith_type=Boolean  n_bits=16  bin_pt=1  preci_type=Single  exp_width=8  frac_width=24  explicit_period=off  period=1  XmcBlockStatus=1  maskContainerNames=tabcontainer1  block_type=constant  block_config=sysgen:Constant_config
  Mux1 : hdlBasic/Mux  inputs=2  en=off  latency=0  precision=Full  arith_type=Unsigned  n_bits=16  bin_pt=14  quantization=Truncate  overflow=Wrap  XmcBlockStatus=1  maskContainerNames=tabcontainer1  block_type=mux  block_config=sysgen:Mux_config
  Register1 : hdlBasic/Register  init=0  rst=on  en=on  XmcBlockStatus=1  maskContainerNames=tabcontainer1  block_type=register  block_config=sysgen:Register_config
  Relational2 : hdlBasic/Relational  mode=a>b  op_type=Bool  en=off  latency=0  XmcBlockStatus=1  maskContainerNames=tabcontainer1  block_type=relational  block_config=sysgen:Relational_config
  Relational3 : hdlBasic/Relational  mode=a>b  op_type=Bool  en=off  latency=0  XmcBlockStatus=1  maskContainerNames=tabcontainer1  block_type=relational  block_config=sysgen:Relational_config
  reg_o : Outport
  wires:
  Constant5/1 -> Accumulator1/1
  Relational2/1 -> Mux1/2
  Constant7/1 -> Mux1/3
  reg_i/1 -> Absolute1/1, Register1/1
  rst/1 -> Register1/2, Accumulator1/2
  Constant6/1 -> Relational3/2
  Accumulator1/1 -> Relational3/1
  Relational3/1 -> Mux1/1
  Mux1/1 -> Register1/3, Accumulator1/3
  Absolute1/1 -> Relational2/1
  Constant4/1 -> Relational2/2
  Register1/1 -> reg_o/1

== system Arm_core_design_block/Subsystem11/Subsystem14 ==
  rst : Inport
  reg_i : Inport  Port=2
  Absolute1 : hdlBasic/Absolute  precision=User Defined  arith_type="Signed  (2's comp)"  n_bits=16  bin_pt=13  quantization=Truncate  overflow=Saturate  en=off  latency=0  XmcBlockStatus=1  maskContainerNames=tabcontainer1  block_type=abs  block_config=sysgen:Abs_config
  Accumulator1 : hdlBasic/Accumulator  operation=Add  n_bits=16  overflow=Wrap  scale=1  rst=on  hasbypass=off  en=on  latency=1  msb_inp=100  msb=100  lsb=-100  use_behavioral_HDL=on  implementation=Fabric  XmcBlockStatus=1  maskContainerNames=group3  block_type=accum  block_config=sysgen:Accum_config
  Constant4 : hdlBasic/Constant  const=0.05  gui_display_data_type=Fixed-point  arith_type=Signed (2's comp)  n_bits=16  bin_pt=14  preci_type=Single  exp_width=8  frac_width=24  explicit_period=off  period=1  XmcBlockStatus=1  maskContainerNames=tabcontainer1  block_type=constant  block_config=sysgen:Constant_config
  Constant5 : hdlBasic/Constant  const=1  gui_display_data_type=Fixed-point  arith_type=Unsigned  n_bits=16  bin_pt=1  preci_type=Single  exp_width=8  frac_width=24  explicit_period=off  period=1  XmcBlockStatus=1  maskContainerNames=tabcontainer1  block_type=constant  block_config=sysgen:Constant_config
  Constant6 : hdlBasic/Constant  const=0  gui_display_data_type=Fixed-point  arith_type=Unsigned  n_bits=16  bin_pt=1  preci_type=Single  exp_width=8  frac_width=24  explicit_period=off  period=1  XmcBlockStatus=1  maskContainerNames=tabcontainer1  block_type=constant  block_config=sysgen:Constant_config
  Constant7 : hdlBasic/Constant  const=0  gui_display_data_type=Boolean  arith_type=Boolean  n_bits=16  bin_pt=1  preci_type=Single  exp_width=8  frac_width=24  explicit_period=off  period=1  XmcBlockStatus=1  maskContainerNames=tabcontainer1  block_type=constant  block_config=sysgen:Constant_config
  Mux1 : hdlBasic/Mux  inputs=2  en=off  latency=0  precision=Full  arith_type=Unsigned  n_bits=16  bin_pt=14  quantization=Truncate  overflow=Wrap  XmcBlockStatus=1  maskContainerNames=tabcontainer1  block_type=mux  block_config=sysgen:Mux_config
  Register1 : hdlBasic/Register  init=0  rst=on  en=on  XmcBlockStatus=1  maskContainerNames=tabcontainer1  block_type=register  block_config=sysgen:Register_config
  Relational2 : hdlBasic/Relational  mode=a>b  op_type=Bool  en=off  latency=0  XmcBlockStatus=1  maskContainerNames=tabcontainer1  block_type=relational  block_config=sysgen:Relational_config
  Relational3 : hdlBasic/Relational  mode=a>b  op_type=Bool  en=off  latency=0  XmcBlockStatus=1  maskContainerNames=tabcontainer1  block_type=relational  block_config=sysgen:Relational_config
  reg_o : Outport
  wires:
  Constant5/1 -> Accumulator1/1
  Relational2/1 -> Mux1/2
  Constant7/1 -> Mux1/3
  reg_i/1 -> Absolute1/1, Register1/1
  rst/1 -> Register1/2, Accumulator1/2
  Constant6/1 -> Relational3/2
  Accumulator1/1 -> Relational3/1
  Relational3/1 -> Mux1/1
  Mux1/1 -> Register1/3, Accumulator1/3
  Absolute1/1 -> Relational2/1
  Constant4/1 -> Relational2/2
  Register1/1 -> reg_o/1
